simulink model "lift_hierarchy"  (R2020a)
settings: Solver=VariableStepAuto  StartTime=0.0  StopTime=10.0  RelTol=1e-3
settings Model: Creator=kiran  LastModifiedBy=kiran

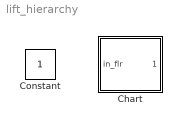
== system lift_hierarchy ==
  Chart : Stateflow chart  TreatAsAtomicUnit=on
  Constant : Constant

== stateflow chart lift_hierarchy/Chart ==
  state Active_state
    state down
      en:
      crnt_flr=crnt_flr-1;
      out_flr=crnt_flr;
    state up
      en:
      crnt_flr=crnt_flr+1;
      out_flr=crnt_flr;
    state stop
      en:
      out_flr=crnt_flr
    stop -> stop [order 3] : [crnt_flr==in_flr]
    (default) -> stop
    up -> stop : [crnt_flr==in_flr]
    stop -> down [order 2] : [crnt_flr>in_flr]
    down -> stop : [crnt_flr==in_flr]
    stop -> up [order 1] : [crnt_flr<in_flr]
  state Same_floor
    en:
    count=0;
    during:
    count=count+1;
  (default) -> Active_state
  (junction 7) -> stop [order 1]
  (junction 7) -> up [order 3] : [crnt_flr<in_flr]
  (junction 7) -> down [order 2] : [crnt_flr>in_flr]
  Active_state -> Same_floor : [crnt_flr==in_flr]
  Same_floor -> (junction 7) : [count==5]
  data: in_flr input; out_flr output; count local =0; crnt_flr local =0
